simulink model "batteryNASAslx"  (R2019a)
settings: Solver=VariableStepAuto  StartTime=0.0  StopTime=300  RelTol=1e-3
InitFcn:
  | %load('batteryModelNew.mat');
  | %load('soc_ocv_new.mat');
  | load('currentUAV.mat');
  | 
  | 
  | battery = BatteryCircuit.Create;
  | 
  | Tb0 = battery.states(1).x0;
  | qb0 = battery.states(2).x0;
  | qcp0 = battery.states(3).x0;
  | qcs0 = battery.states(4).x0;
  | 
  | parameters = battery.P;
  | 
  | V0 = parameters.V0;
  | Rp = parameters.Rp;
  | qMax = parameters.qMax;
  | CMax = parameters.CMax;
  | Cb0 = parameters.Cb0;
  | Cbp0 = parameters.Cbp0;
  | Cbp1 = parameters.Cbp1;
  | Cbp2 = parameters.Cbp2;
  | Cbp3 = parameters.Cbp3;
  | Rs = parameters.Rs;
  | Cs = parameters.Cs;
  | Rcp0 = parameters.Rcp0;
  | Rcp1 = parameters.Rcp1;
  | Rcp2 = parameters.Rcp2;
  | Ccp = parameters.Ccp;
  | Ta = parameters.Ta;
  | Jt = parameters.Jt;
  | ha = parameters.ha;
  | hcp = parameters.hcp;
  | hcs = parameters.hcs;
  | VEOD = parameters.VEOD;
libraries: dspsrcs4 x1
settings Model: Creator=tdarrah  LastModifiedBy=tdarrah
settings DebuggingCC: UnderSpecifiedDimensionMsg=warning

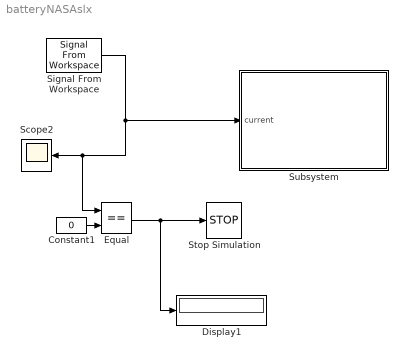
== system batteryNASAslx ==
  Constant1 : Constant  Value=0
  Display1 : Display
  Equal : RelationalOperator  Operator===  OutDataTypeStr=boolean  RndMeth=Simplest
  Scope2 : Scope
  Signal From Workspace : dspsrcs4/Signal From Workspace  X=current  Ts=1/36  nsamps=1  OutputAfterFinalValue=Setting to zero  ignoreOrWarnInputAndFrameLengths=off  OutputFrames=off
  Stop Simulation : Stop
  Subsystem : Subsystem
  wires:
  Signal From Workspace/1 -> Equal/1, Scope2/1, Subsystem/1(current)
  Constant1/1 -> Equal/2
  Equal/1 -> Display1/1, Stop Simulation/1

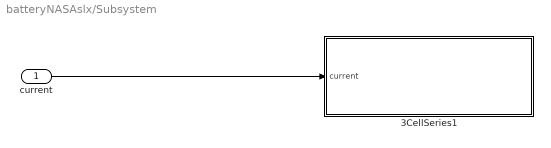
== system batteryNASAslx/Subsystem ==
  current : Inport
  3CellSeries1 : Subsystem
  wires:
  current/1 -> 3CellSeries1/1(current)

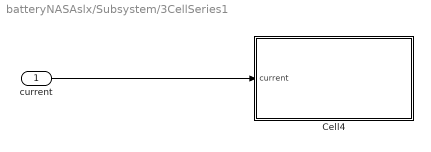
== system batteryNASAslx/Subsystem/3CellSeries1 ==
  current : Inport
  Cell4 : Subsystem
  wires:
  current/1 -> Cell4/1(current)

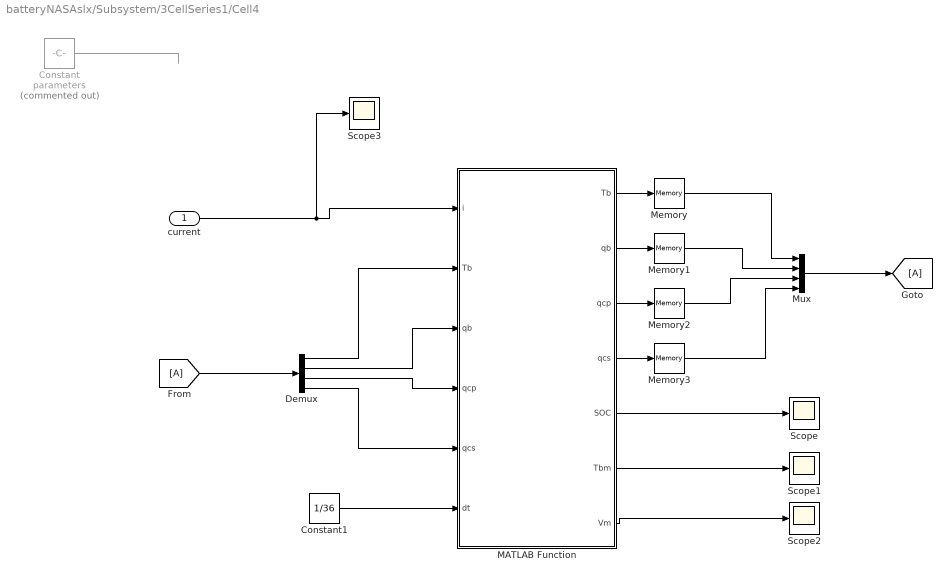
== system batteryNASAslx/Subsystem/3CellSeries1/Cell4 ==
  current : Inport
  Constant : Constant  Commented=on  Value=parameters
  Constant1 : Constant  Value=1/36
  Demux : Demux
  MATLAB Function : MATLAB Function  TreatAsAtomicUnit=on
  Memory{,1..3} (4 alike) : Memory  InitialCondition=Tb0  InheritSampleTime=on  LinearizeAsDelay=on
  Mux : Mux
  Scope{,1..3} (4 alike) : Scope
  wires:
  current/1 -> Scope3/1, MATLAB Function/1(i)
  MATLAB Function/1(Tb) -> Memory/1
  MATLAB Function/2(qb) -> Memory1/1
  MATLAB Function/3(qcp) -> Memory2/1
  MATLAB Function/4(qcs) -> Memory3/1
  Mux/1 -> [A]
  [A] -> Demux/1
  Demux/1 -> MATLAB Function/2("Tb ")
  Demux/2 -> MATLAB Function/3("qb ")
  Demux/3 -> MATLAB Function/4("qcp ")
  Demux/4 -> MATLAB Function/5("qcs ")
  Memory/1 -> Mux/1
  Memory1/1 -> Mux/2
  Memory2/1 -> Mux/3
  Memory3/1 -> Mux/4
  MATLAB Function/5(SOC) -> Scope/1
  MATLAB Function/6(Tbm) -> Scope1/1
  MATLAB Function/7(Vm) -> Scope2/1
  Constant1/1 -> MATLAB Function/6(dt)
  Constant/1 -> ?

== matlab function batteryNASAslx/Subsystem/3CellSeries1/Cell4/MATLAB Function ==
  data: Tb output; i input; Tb input; qb output; qcp output; qcs output; qb input; qcp input; qcs input; dt input; SOC output; Tbm output; Vm output
function [Tb, qb, qcp, qcs, SOC, Tbm, Vm]= StateEqn(i, Tb, qb, qcp, qcs, dt)
    SOC = 0.0;
    Tbm = 0.0;
    Vm = 0.0;
    
    parameters.Rp = 10000;
    parameters.qMax = 7.8563e+03;
    parameters.CMax = 7777;
    parameters.Cb0 = 1.8782e+03;
    parameters.Cbp0= -230;
    parameters.Cbp1= 1.2000;
    parameters.Cbp2= 2.0799e+03;
    parameters.Cbp3= 27.0557;
    parameters.Rs= 0.0539;
    parameters.Cs= 234.3870;
    parameters.Rcp0= 0.0698;
    parameters.Rcp1= 1.5053e-17;
    parameters.Rcp2= 37.2230;
    parameters.Ccp= 14.8223;
    parameters.Ta= 18.9500;
    parameters.Jt= 800;
    parameters.ha= 0.5000;
    parameters.hcp= 19;
    parameters.hcs= 1;
    

    Vcs = qcs./parameters.Cs;
    Vcp = qcp./parameters.Ccp;
    SOC = (parameters.CMax - parameters.qMax + qb)./parameters.CMax;
    Cb = parameters.Cbp0.*SOC.^3 + parameters.Cbp1.*SOC.^2 + parameters.Cbp2.*SOC + parameters.Cbp3;
    Rcp = parameters.Rcp0 + parameters.Rcp1.*exp(parameters.Rcp2.*(-SOC + 1));
    Vb = qb./Cb;
    Tbdot = (Rcp.*parameters.Rs.*parameters.ha.*(parameters.Ta - Tb) + Rcp.*Vcs.^2.*parameters.hcs + parameters.Rs.*Vcp.^2.*parameters.hcp)./(parameters.Jt.*Rcp.*parameters.Rs);
    Vp = Vb - Vcp - Vcs;
    ip = Vp./parameters.Rp;
    ib = i + ip;
    icp = ib - Vcp./Rcp;
    qcpdot = icp;
    qbdot = -ib;
    ics = ib - Vcs./parameters.Rs;
    qcsdot = ics;
    
    Tb = Tb + Tbdot*dt;
    qb = qb + qbdot*dt;
    qcp = qcp + qcpdot*dt;
    qcs = qcs + qcsdot*dt;
    
    Tbm = Tb;
    Vm = Vp;
